simulink model "Copy_of_MPC_control"  (R2018a)
settings: Solver=FixedStepAuto  StartTime=0  StopTime=Tend  FixedStep=0.001  RelTol=5e-3
model workspace (MAT data in the model file):
  A_mu = 10
  B_reff = 8.386
  Cz = 7766.25
  DCT_Param : struct (value not decoded)
  D_reff = 0.25826
  Downshift_Speeds = [9.5625 12.9375 16.3125 19.6875 23.0625 26.4375 29.8125 33.1875 36.5625 39.9375 43.3125 46.6875 ... (28 elements, 4x7)]
  Pedal_Positions = [0.1 0.4 0.5 0.9]
  SUS : struct (value not decoded)
  Upshift_Speeds = [12.9375 16.3125 19.6875 33 26.4375 29.8125 33.1875 52.5 39.9375 43.3125 46.6875 77.25 ... (28 elements, 4x7)]
  VEH : struct (value not decoded)
  V_o = 16.7
  V_xlow = 1
  WH : struct (value not decoded)
  a = 1.4
  alpha_max = 1.5
  alpha_min = -1.5
  b = 1.8
  c_zo = 209651
  epsilon = 0.1
  h = 0.134
  path : struct (value not decoded)
  pio = 220000
  q_Fcx = 0
  q_Fz2 = 15.4
  q_Fzy = 0
  q_reo = 0.9974
  q_sx1 = -0.007764
  q_sx10 = 0.2824
  q_sx11 = 5.349
  q_sx12 = 0
  q_sx13 = 0
  q_sx14 = 0
  q_sx2 = 1.1915
  q_sx3 = 0.013948
  q_sx4 = 4.912
  q_sx5 = 1.02
  q_sx6 = 22.83
  q_sx7 = 0.7104
  q_sx8 = -0.023393
  q_sx9 = 0.6581
  q_sy1 = 0.00702
  q_sy2 = 0
  q_sy3 = 0.001515
  q_sy4 = 8.514e-05
  q_sy5 = 0
  q_sy6 = 0
  q_sy7 = 0.9008
  q_sy8 = -0.4089
  q_v1 = 0.0007742
  q_v2 = 0.04667
  r_Bx1 = 12.531
  r_Bx2 = 9.532
  r_Bx3 = 0
  r_By1 = 10.615
  r_By2 = 7.705
  r_By3 = 3.433e-06
  r_By4 = 0
  r_Cx1 = 1.019
  r_Cy1 = 1.0585
  r_Ex1 = -0.4487
  r_Ex2 = -0.4726
  r_Ey1 = 0.3132
  r_Ey2 = 7.63e-06
  r_Hx1 = 0.0002374
  r_Hy1 = 0.011646
  r_Hy2 = 7.63e-06
  r_Vy1 = 0.05654
  r_Vy2 = 7.63e-06
  r_Vy3 = 0
  r_Vy4 = 99.9
  r_Vy5 = 2
  r_Vy6 = 15.814
  r_o = 0.3135
  vehWidth = 2
  w = 1
symbols that are objects in the model workspace (value not decoded): VEH
undefined symbols (not defined in the file): C_Brake, C_Final, C_Front, C_Front_1, C_Front_2, C_Middle, C_out_Brake, C_out_Final, C_out_Front, C_out_Front_1, C_out_Front_2, C_out_Middle, Co, Cok_Brake, Cok_Final, Cok_Front_1, Cok_Front_2, Cok_Middle, Cso, D_out_Brake, D_out_Final, D_out_Front, D_out_Front_1, D_out_Front_2, D_out_Middle, Earlytochange, Earlytochange2, F, F_Brake, F_Final, F_Front, F_Front_1, F_Front_2, F_Middle, Fs, G_Brake, G_Final, G_Front_1, G_Front_2, G_Middle, G_sys_Brake, G_sys_Final, G_sys_Front, G_sys_Front_1, G_sys_Front_2, G_sys_Middle, Gd, Gd_Brake, Gd_Final, Gd_Front, Gd_Front_1, Gd_Front_2, Gd_Middle, Go, Gsd, Gso, H_Brake, H_Final, H_Front_1, H_Front_2 ... (+60)
libraries: simulink x10, sim3dlib x4, autolibutils x2, vehdynlibviscommon x2
(part 7 of 8)

== matlab function Copy_of_MPC_control/observer/simulator_1/VH2P/YV2P ==
  data: Velocity input; LastVelocity input; Yaw input; LastYaw input; Tsim input; LastTsim input; Lastpostion input; Position output
function Position  = YV2P(Velocity,LastVelocity, Yaw, LastYaw, Tsim, LastTsim, Lastpostion)
if Tsim >= 0.1
    Position = zeros(2,1);
    X0 = Lastpostion(1,:); Y0 = Lastpostion(2,:);
    Vx0 = [LastVelocity*cos(LastYaw); Velocity*cos(Yaw)];
    Vy0 = [LastVelocity*sin(LastYaw); Velocity*sin(Yaw)];
    Yaw_sim = [LastYaw; Yaw];
    T =[LastTsim; Tsim];
    [ X_tmp, Y_tmp] = YV2P( T, X0, Y0, Vx0, Vy0, Yaw_sim, zeros(2,1) );
    Position = [X_tmp(end,:); Y_tmp(end,:)];
else
    Position = [0; 0];
end
end

== matlab function Copy_of_MPC_control/observer/observer_2/gate ==
  data: select_overlap input; state output
function state = gate(select_overlap)
if select_overlap == 2
    state = 1;
else
    state = 0;
end
end

== matlab function Copy_of_MPC_control/observer/simulator_3/VH2P/YV2P ==
  data: Velocity input; LastVelocity input; Yaw input; LastYaw input; Tsim input; LastTsim input; Lastpostion input; Position output
function Position  = YV2P(Velocity,LastVelocity, Yaw, LastYaw, Tsim, LastTsim, Lastpostion)
if Tsim >= 0.1
    Position = zeros(2,1);
    X0 = Lastpostion(1,:); Y0 = Lastpostion(2,:);
    Vx0 = [LastVelocity*cos(LastYaw); Velocity*cos(Yaw)];
    Vy0 = [LastVelocity*sin(LastYaw); Velocity*sin(Yaw)];
    Yaw_sim = [LastYaw; Yaw];
    T =[LastTsim; Tsim];
    [ X_tmp, Y_tmp] = YV2P( T, X0, Y0, Vx0, Vy0, Yaw_sim, zeros(2,1) );
    Position = [X_tmp(end,:); Y_tmp(end,:)];
else
    Position = [0; 0];
end
end

== matlab function Copy_of_MPC_control/observer/simulator_2/Mpc_Simulator_Middle/MATLAB Function ==
  data: r output; JE input; phi input; Fxh input; Qc input; U output; M input; Np input; Heading_updated input; Velocity_updated input; Rs input; Tsim input; select_MPC input; U_delay input
function [r,U] = HQP(JE ,phi,Fxh ,Qc ,M ,Np,Heading_updated ,Velocity_updated ,Rs ,Tsim, select_MPC,U_delay)
u1_max =  5/3*pi; u1_min = -5/3*pi;
u2_max =  1; u2_min = -1;
du1_inc =  1*5/3*pi;du1_dec =  1*5/3*pi;
du2_inc =  1;du2_dec =  1;
U_max = []; U_min = [];
for i = 1:Np
    U_max = [U_max; [u1_max; u2_max]];
    U_min = [U_min; [-u1_min; -u2_min]];
end

dU_plus = []; dU_minus = [];
for i = 1:Np
    dU_plus = [dU_plus; [U_delay(1) + du1_inc; U_delay(2) + du2_inc]];
    dU_minus = [dU_minus; [-U_delay(1) + du1_dec; -U_delay(2) + du2_dec;]];
end
N = [U_max;
      U_min;
      dU_plus;
      dU_minus;          
     ];
if Tsim > 0 && select_MPC ~= 5
    for i = 1: Np
        Rs(2*i,:) = Heading_updated(i,:);
        Rs(2*i-1,:) = Velocity_updated(i,:);
    end
end
JF = -2*phi'*Qc*(Rs-Fxh);
[u,lambda]= HQP(JE,JF,M,N);
U = u(1:2);
r = Rs(1:2,:);
end

== matlab function Copy_of_MPC_control/YV_update/MATLAB Function2 ==
  data: XYplot_ref input; Velocity_updated output; XYplot_sim input; Velocity_sim input; Yaw_sim input; Ts input; Tsim input; Heading_updated output
function [Velocity_updated, Heading_updated] = VY_update(XYplot_ref, XYplot_sim, Velocity_sim, Yaw_sim, Ts, Tsim)
Np = 6;
Heading_updated = zeros(Np,1); Velocity_updated = zeros(Np,1);
coder.extrinsic('P2YV');
T = []; 
for j = 1:Np+1
    T = [T; Tsim+(j-1)*Ts];
end
X = [];
for i = 1:Np
    X = [X; XYplot_ref(2*i-1,:)];
end
Y = [];
for i = 1:Np
    Y = [Y; XYplot_ref(2*i,:)];
end

X = [XYplot_sim(1,:); X];
Y = [XYplot_sim(2,:); Y];   
Vx0 = Velocity_sim*cos(Yaw_sim);
Vy0 = Velocity_sim*sin(Yaw_sim);
Yaw0 = Yaw_sim;

[Velocity_updated, Heading_updated] = P2YV(0,0, T , X , Y , Vx0 , Vy0 , Yaw0, Np, 0, 0 );
end

== matlab function Copy_of_MPC_control/observer/simulator_2/VH2P/YV2P ==
  data: Velocity input; LastVelocity input; Yaw input; LastYaw input; Tsim input; LastTsim input; Lastpostion input; Position output
function Position  = YV2P(Velocity,LastVelocity, Yaw, LastYaw, Tsim, LastTsim, Lastpostion)
if Tsim >= 0.1
    Position = zeros(2,1);
    X0 = Lastpostion(1,:); Y0 = Lastpostion(2,:);
    Vx0 = [LastVelocity*cos(LastYaw); Velocity*cos(Yaw)];
    Vy0 = [LastVelocity*sin(LastYaw); Velocity*sin(Yaw)];
    Yaw_sim = [LastYaw; Yaw];
    T =[LastTsim; Tsim];
    [ X_tmp, Y_tmp] = YV2P( T, X0, Y0, Vx0, Vy0, Yaw_sim, zeros(2,1) );
    Position = [X_tmp(end,:); Y_tmp(end,:)];
else
    Position = [0; 0];
end
end

== matlab function Copy_of_MPC_control/observer/simulator_2/VH2P/gate ==
  data: select_overlap input; state output
function state = gate(select_overlap)
if select_overlap == 2
    state = 1;
else
    state = 0;
end
end

== matlab function Copy_of_MPC_control/Controllers/ECU/MATLAB Function ==
  data: input output; input input; output output
function [input,output] = debug(input)
if isnan(input) || isinf(input)
    output = 1;
    input = 0;
else
    output = 0;
    input = input;
end
end

== matlab function Copy_of_MPC_control/observer123/Final Observer2/Subsystem/Mpc_Simulator_Final/MATLAB Function ==
  data: Upd_flag input; Timetochange input; Ref output; JE input; U output; M input; Np input; phi input; Qc input; Fxh input; Yup input; Vup input; Rs input; Rs_V input; Tsim input; Upd_end input; u input
function [Ref,U] = HQP(Upd_flag, Timetochange,JE,M,Np,phi,Qc,Fxh,Yup,Vup,Rs,Rs_V,Tsim,Upd_end,u)

% if Tsim < 6.27 %(sec)
%     u1_max =  5/3*pi; u1_min = -5/3*pi;
%     u2_max =  0.3; u2_min = -1;
%     du1_inc =  1*5/3*pi; 
%     du1_dec =  1*5/3*pi; 
%     du2_inc =  0.03;
%     du2_dec =  0.03;
% else 
    u1_max =  5/3*pi; u1_min = -5/3*pi;
    u2_max =  1; u2_min = -1;
    du1_inc =  1*5/3*pi;
    du1_dec =  1*5/3*pi;
    du2_inc =  1;
    du2_dec =  1;
% end
% du1_max =  0.1*abs(Fxh(1,:)); 
% du2_max =  0.05*abs(Fxh(1,:)); 
% Y1_min = Rs(1,:) - 2;%V
% Y1_max = Rs(1,:) + 2;%V
% Y2_min = Rs(2,:) - 0.2;%Y
% Y2_max = Rs(2,:) + 0.2;%Y
% 
% Y1_min = -10;%V
% Y2_min = -100;%Y
% Y1_max = 50;%V
% Y2_max = 100;%Y

% Y_max = [];
% Y_min = [];
% for i = 1:Np
%     Y_max = [Y_max;[Y1_max;Y2_max]];
%     Y_min = [Y_min;[Y1_min;Y2_min]];
% end

U_max = []; U_min = [];
for i = 1:Np
    U_max = [U_max; [u1_max; u2_max]];
    U_min = [U_min; [-u1_min; -u2_min]];
end

dU_plus = []; dU_minus = [];
for i = 1:Np
    dU_plus = [dU_plus; [u(1) + du1_inc; u(2) + du2_inc]];
    dU_minus = [dU_minus; [-u(1) + du1_dec; -u(2) + du2_dec;]];
end
rr = [U_max;
      U_min;
      dU_plus;
      dU_minus;          
     ];
 
% rr_y = [Y_max - Fxh;
%        -Y_min + Fxh;
%        ];
N = [];
N = rr; 
% N = [rr;rr_y];


if Tsim > 0 && Tsim < Upd_end
    for i = 1: Np
        Rs(2*i,:) = Yup(i,:);
        Rs(2*i-1,:) = Vup(i,:);
    end
% elseif Tsim >= 65
%     for i = 1: Np
%         Rs(2*i,:) = Yup(i,:);
% %         Rs(2*i-1,:) = Vup(i,:);
%     end
end


JF = -2*phi'*Qc*(Rs-Fxh);
[uc,lambda]= HQP(JE,JF,M,N);
U = uc(1:2);
% if Tsim <= Timetochange
%     U(1,:) = 1e-9;
% end
Ref = Rs(1:2,:);
% lambda
end

== matlab function Copy_of_MPC_control/observer/simulator_2/YV_update_Np/MATLAB Function2 ==
  data: XYplot_ref input; Velocity_updated output; XYplot_sim input; Velocity_sim input; Yaw_sim input; Ts input; Tsim input; Heading_updated output
function [Velocity_updated, Heading_updated] = VY_update(XYplot_ref, XYplot_sim, Velocity_sim, Yaw_sim, Ts, Tsim)
Np = 6;
 disp(sprintf('Simulation time : %2.1f sec',Tsim)) 
 Heading_updated = zeros(Np,1); Velocity_updated = zeros(Np,1);
coder.extrinsic('P2YV');
T = []; 
for j = 1:Np+1
    T = [T; Tsim+(j-1)*Ts];
end
X = [];
for i = 1:Np
    X = [X; XYplot_ref(2*i-1,:)];
end
Y = [];
for i = 1:Np
    Y = [Y; XYplot_ref(2*i,:)];
end

X = [XYplot_sim(1,:); X];
Y = [XYplot_sim(2,:); Y];   
Vx0 = Velocity_sim*cos(Yaw_sim);
Vy0 = Velocity_sim*sin(Yaw_sim);
Yaw0 = Yaw_sim;

[Velocity_updated, Heading_updated] = P2YV(0,0, T , X , Y , Vx0 , Vy0 , Yaw0, Np, 0, 0 );
end

== matlab function Copy_of_MPC_control/observer/simulator_2/gate ==
  data: select_overlap input; state output
function state = gate(select_overlap)
if select_overlap == 2
    state = 1;
else
    state = 0;
end
end

== stateflow chart Copy_of_MPC_control/all_system/Controllers1/Transmission Controller/TCM/TCM Shift Controller ==
  settings: sampleTime=0.01
  state GearState [parallel]
    settings: executionOrder=1
    state Neutral
      en:
      GearState = 0;
    state G1
      en:
      GearState = 1;
    state G2
      en:
      GearState = 2;
      du:
      [SpdThr] = calc(2,pedal,speed);
    state G3
      en:
      GearState = 3;
      du:
      [SpdThr] = calc(3,pedal,speed);
    state G8
      en:
      GearState = 8;
    state G7
      en:
      GearState = 7;
    state G6
      en:
      GearState = 6;
    state G5
      en:GearState=5;
      du:[SpdThr]=calc(5,pedal,speed);
    state G4
      en:
      GearState = 4;
      du:
      [SpdThr] = calc(4,pedal,speed);
    (default) -> G1
    Neutral -> G1 : [~Neutral]
    G1 -> G2 [order 1] : Up
    G2 -> G3 [order 1] : Up
    G1 -> Neutral [order 2] : [Neutral]
    G2 -> G1 [order 2] : Down
    G3 -> G2 [order 2] : Down
    G3 -> G4 [order 1] : Up
    G4 -> G3 [order 2] : Down
    G7 -> G8 [order 1] : Up
    G5 -> G6 [order 1] : Up
    G6 -> G7 [order 1] : Up
    G4 -> G5 [order 1] : Up
    G5 -> G4 [order 2] : Down
    G6 -> G5 [order 2] : Down
    G7 -> G6 [order 2] : Down
    G8 -> G7 : Down
  state SelectionState [parallel]
    du:[up_th]=calc_up(GearState,pedal);
    du:[down_th]=calc_down(GearState,pedal);
    settings: executionOrder=2
    state SteadyState
      en:
      clutchControl = 0;
    state preDownShifting
    state preUpShifting
    state UpShifting
      en:
      GearState = GearState + 0.5;
    state DownShifting
      en:
      GearState = GearState - 0.5;
    (default) -> SteadyState
    SteadyState -> (junction 62) [order 1] : [speed < down_th && ...
        | GearState >1]
    SteadyState -> (junction 128) [order 2] : [speed > up_th &&...
        | GearState <= 5 && ...
        | floor(GearState) == GearState]
    (junction 62) -> preDownShifting
    (junction 128) -> preUpShifting
    (junction 168) -> SteadyState
    (junction 23) -> SteadyState
    (junction 161) -> SteadyState
    preDownShifting -> (junction 168) [order 2] : [speed >= down_th]
    preUpShifting -> (junction 161) [order 2] : [speed <= up_th]
    preUpShifting -> UpShifting [order 1] : after(0.5,sec)
        | [speed>up_th]
    preDownShifting -> DownShifting [order 1] : after(0.5, sec)
        | [speed < down_th - 2]
    DownShifting -> (junction 23) : {GearState.Down;}
    UpShifting -> (junction 23) : {GearState.Up;}
  state up_th = calc_up(gear,pedal) [function]
  state down_th = calc_down(gear,pedal) [function]
  state SpdThr = calc(gear,pedal,speed) [function]
  data: gear function_input; pedal function_input; up_th function_output; gear function_input; pedal function_input; down_th function_output; gear function_input; pedal function_input; SpdThr function_output; speed function_input; GearState output int8; speed input; pedal input; clutchControl local double; SpdThr local double; Neutral input; up_th local double; down_th local double
  events: Up local EITHER_EDGE_EVENT; Down local EITHER_EDGE_EVENT

== matlab function Copy_of_MPC_control/all_system/Dataselect1/Dataselect ==
  data: timing input; select output; Statechange input; Statechange2 input
function select = Dataselect(timing,Statechange,Statechange2)    
    if timing < Statechange
        select = 1;
    elseif timing < Statechange2
        select = 2;
    else 
        select = 3;
    end
end

== matlab function Copy_of_MPC_control/all_system/Final Observer2/Subsystem/Mpc_Simulator_Final/MATLAB Function ==
  data: Upd_flag input; Timetochange input; Ref output; JE input; U output; M input; Np input; phi input; Qc input; Fxh input; Yup input; Vup input; Rs input; Rs_V input; Tsim input; Upd_end input; u input
function [Ref,U] = HQP(Upd_flag, Timetochange,JE,M,Np,phi,Qc,Fxh,Yup,Vup,Rs,Rs_V,Tsim,Upd_end,u)

% if Tsim < 6.27 %(sec)
%     u1_max =  5/3*pi; u1_min = -5/3*pi;
%     u2_max =  0.3; u2_min = -1;
%     du1_inc =  1*5/3*pi; 
%     du1_dec =  1*5/3*pi; 
%     du2_inc =  0.03;
%     du2_dec =  0.03;
% else 
    u1_max =  5/3*pi; u1_min = -5/3*pi;
    u2_max =  1; u2_min = -1;
    du1_inc =  1*5/3*pi;
    du1_dec =  1*5/3*pi;
    du2_inc =  1;
    du2_dec =  1;
% end
% du1_max =  0.1*abs(Fxh(1,:)); 
% du2_max =  0.05*abs(Fxh(1,:)); 
% Y1_min = Rs(1,:) - 2;%V
% Y1_max = Rs(1,:) + 2;%V
% Y2_min = Rs(2,:) - 0.2;%Y
% Y2_max = Rs(2,:) + 0.2;%Y
% 
% Y1_min = -10;%V
% Y2_min = -100;%Y
% Y1_max = 50;%V
% Y2_max = 100;%Y

% Y_max = [];
% Y_min = [];
% for i = 1:Np
%     Y_max = [Y_max;[Y1_max;Y2_max]];
%     Y_min = [Y_min;[Y1_min;Y2_min]];
% end

U_max = []; U_min = [];
for i = 1:Np
    U_max = [U_max; [u1_max; u2_max]];
    U_min = [U_min; [-u1_min; -u2_min]];
end

dU_plus = []; dU_minus = [];
for i = 1:Np
    dU_plus = [dU_plus; [u(1) + du1_inc; u(2) + du2_inc]];
    dU_minus = [dU_minus; [-u(1) + du1_dec; -u(2) + du2_dec;]];
end
rr = [U_max;
      U_min;
      dU_plus;
      dU_minus;          
     ];
 
% rr_y = [Y_max - Fxh;
%        -Y_min + Fxh;
%        ];
N = [];
N = rr; 
% N = [rr;rr_y];


if Tsim > 0 && Tsim < Upd_end
    for i = 1: Np
        Rs(2*i,:) = Yup(i,:);
        Rs(2*i-1,:) = Vup(i,:);
    end
% elseif Tsim >= 65
%     for i = 1: Np
%         Rs(2*i,:) = Yup(i,:);
% %         Rs(2*i-1,:) = Vup(i,:);
%     end
end


JF = -2*phi'*Qc*(Rs-Fxh);
[uc,lambda]= HQP(JE,JF,M,N);
U = uc(1:2);
% if Tsim <= Timetochange
%     U(1,:) = 1e-9;
% end
Ref = Rs(1:2,:);
% lambda
end

== matlab function Copy_of_MPC_control/all_system/Final Observer2/Subsystem/Pose updete k/Update ==
  settings: updateMethod=DISCRETE  sampleTime=Ts
  data: Rs_V_now input; Rs_Y_now input; XYline input; XYplot input; XYplot_sim input; Last_XYplot_sim input; Velocity_sim input; Last_Velocity_sim input; Heading_sim input; Last_Heading_sim input; Tsim input; Last_Heading_end input; Velocity_updated output; Heading_updated output [1..5]; Heading_end output
function [Velocity_updated, Heading_updated, Heading_end] = Y_update(Rs_V_now, Rs_Y_now, ...
        XYline, XYplot, XYplot_sim, Last_XYplot_sim, Velocity_sim, Last_Velocity_sim, Heading_sim, Last_Heading_sim, ... 
    Tsim, Last_Heading_end)
    disp(sprintf('Simulation time : %2.1f sec',Tsim)) 
    Np = 5; Ts = 0.1;
    Heading_updated = zeros(Np,1); Velocity_updated = zeros(Np,1);Heading_end = 0;
    coder.extrinsic('intersections');
    coder.extrinsic('P2YV');
%     coder.varsize('Velocity_updated_tmp',[5 1]);
%     coder.varsize('Heading_updated_tmp',[5 1]);
     if Tsim == 0 
        plot(XYline(:,2),XYline(:,1),'black');
    end
   

%%Create half-circle    

    N = 30;
    theta = zeros(Np-1,N+1); Veh_circle = zeros(N+1,(Np-1)*2); 
    xp = zeros(1,N+1); yp = zeros(1,N+1); X = [];  Y = []; X_tmp = 0; Y_tmp = 0;
    lookahead = zeros(Np-1,1);
    
    XYplot_sim_tmp = XYplot_sim;    

%     if Velocity_sim > 0.5
        Velocity_ahead = [Velocity_sim; Rs_V_now(2:Np-1,:)];
%     else
%         Velocity_ahead = Rs_V_now;
%     end

    lookahead = Velocity_ahead*Ts;
    Headngahead = [Heading_sim; Rs_Y_now(2:Np-1,:)];
%     lookahead = [1; 1.5; 2; 2.5; 3];
        
    for j = 1:Np-1        
        theta = Headngahead(j,:)-pi/4 : pi/2/N : Headngahead(j,:)+pi/4;
        xp = lookahead(j,:)*cos(theta) + XYplot_sim_tmp(1,:)*ones(1,length(theta));
        yp = lookahead(j,:)*sin(theta) + XYplot_sim_tmp(2,:)*ones(1,length(theta));
        Veh_circle(:,2*j-1:2*j) = [xp' yp'];
       
    %Find the intersection    
         
        [X_tmp, Y_tmp] = intersections(XYplot(:,1), XYplot(:,2), Veh_circle(:,2*j-1), Veh_circle(:,2*j),0); 
        
        if X_tmp == 0 && Y_tmp == 0
%             X = X_tmp(1:j-1,:);
%             Y = Y_tmp(1:j-1,:);
            break;
        end

        X = [X; X_tmp];
        Y = [Y; Y_tmp];   
        XYplot_sim_tmp = [X_tmp; Y_tmp];
        
    end 
    
%%Obtain predict Velocity and Heading angle
   
  
    
    X = [Last_XYplot_sim(1,:); XYplot_sim(1,:); X];
    Y = [Last_XYplot_sim(2,:); XYplot_sim(2,:); Y];
    Vx0 = Last_Velocity_sim*cos(Last_Heading_sim);
    Vy0 = Last_Velocity_sim*sin(Last_Heading_sim);
    Yaw0 = Last_Heading_sim;
     
    T_sample = []; 
    for j = 1:length(X)
        T_sample = [T_sample; Tsim+(j-1)*Ts];
    end
    
   [Velocity_updated, Heading_updated] = P2YV(0, T_sample , X , Y , Vx0 , Vy0 , Yaw0, Np, Last_Heading_end );
   Heading_end = Heading_updated(end,:);

%     Heading_tmp_end = atan2(XYplot(end,2)-XYplot_sim(2,:), XYplot(end,1)-XYplot_sim(1,:));
% 
%     if  ((Heading_tmp_end - Heading_tmp_end_delay) < -5/3*pi) % Angle compensation
%         Heading_flag_end = Heading_flag_end + 1;
%     elseif ((Heading_tmp_end - Heading_tmp_end_delay) > 5/3*pi)
%         Heading_flag_end = Heading_flag_end - 1;
%     end
%     
%     if flag == 1
%         Heading_updated(1:end) = Heading_tmp_end + Heading_flag_end*2*pi;
%     end
%     if Tsim == 1.5
%         figure();
%         plot(XYplot(:,2),XYplot(:,1),'black-');
%         hold on;
%         plot(XYplot_sim(2,:),XYplot_sim(1,:),'b o');
%         plot(Veh_circle(:,2), Veh_circle(:,1),'b-');
%         plot(Veh_circle(:,4), Veh_circle(:,3),'b-');
%         plot(Veh_circle(:,6), Veh_circle(:,5),'b-');
%         plot(Veh_circle(:,8), Veh_circle(:,7),'b-');
%         plot(Veh_circle(:,10), Veh_circle(:,9),'b-');
%         plot(Y, X,'r x');
%     end

end

== matlab function Copy_of_MPC_control/all_system/Final Observer2/Subsystem/VH2P/YV2P ==
  data: Velocity input; Yaw input; LastVelocity input; LastYaw input; Tsim input; LastTsim input; Lastpostion input; Position output
function Position  = YV2P(Velocity, Yaw,  LastVelocity, LastYaw, Tsim, LastTsim, Lastpostion)
if Tsim >= 0.1
    Position = zeros(2,1);
    X0 = Lastpostion(1,:); Y0 = Lastpostion(2,:);
    Vx = [LastVelocity*cos(LastYaw); Velocity*cos(Yaw)];
    Vy = [LastVelocity*sin(LastYaw); Velocity*sin(Yaw)];
    Yaw_sim = [LastYaw; Yaw];
    T_sample =[LastTsim; Tsim];
    [ X_tmp, Y_tmp] = YV2P( T_sample, X0, Y0, Vx, Vy, Yaw_sim, zeros(2,1) );
    Position = [X_tmp(end,:); Y_tmp(end,:)];
else
    Position = [0; 0];
end

end

== matlab function Copy_of_MPC_control/all_system/Final Observer2/Subsystem/YV_update_Np/MATLAB Function2 ==
  data: XY_ref input; Velocity_updated output; XY_sim input; LastXY_sim input; Velocity_sim input; LastVelocity_sim input; Yaw_sim input; LastYaw_sim input; Tsim input; Heading_updated output
function [Velocity_updated, Heading_updated] = VY_update(XY_ref, XY_sim, LastXY_sim, Velocity_sim, LastVelocity_sim, Yaw_sim, LastYaw_sim, Tsim)
    disp(sprintf('Simulation time : %2.1f sec',Tsim)) 
 Ts = 0.1;
% Np = 6;
 Np = 6;

 Heading_updated = zeros(Np,1); Velocity_updated = zeros(Np,1);
coder.extrinsic('P2YV');
% T_sample = [Tsim-0.01; Tsim; Tsim+0.01];
% X = [LastXY_sim(1); XY_sim(1); XY_ref(1,:)];
% Y = [LastXY_sim(2); XY_sim(2); XY_ref(2,:)];

% T_sample = [Tsim-0.01; Tsim; Tsim+0.01; Tsim+0.02];
% X = [LastXY_sim(1); XY_sim(1); XY_ref(1,:); XY_ref(3,:)];
% Y = [LastXY_sim(2); XY_sim(2); XY_ref(2,:); XY_ref(4,:)];

T_sample = []; 
for j = 1:Np+1
    T_sample = [T_sample; Tsim+(j-1)*Ts];
end
X = [];
for i = 1:Np
    X = [X; XY_ref(2*i-1,:)];
end
Y = [];
for i = 1:Np
    Y = [Y; XY_ref(2*i,:)];
end

X = [XY_sim(1,:); X];
Y = [XY_sim(2,:); Y];   
Vx0 = Velocity_sim*cos(Yaw_sim);
Vy0 = Velocity_sim*sin(Yaw_sim);
Yaw0 = Yaw_sim;

[Velocity_updated, Heading_updated] = P2YV(0,0, T_sample , X , Y , Vx0 , Vy0 , Yaw0, Np, 0, 0 );

end

== matlab function Copy_of_MPC_control/all_system/Final_simulator1/Mpc_Simulator_Final/MATLAB Function ==
  data: Ref output; JE input; U output; M input; Np input; phi input; Qc input; Fxh input; Yup input; Vup input; Rs input; Rs_V input; Tsim input; Upd_end input; u input; lambda output
function [Ref,U,lambda] = HQP(JE,M,Np,phi,Qc,Fxh,Yup,Vup,Rs,Rs_V,Tsim,Upd_end,u)

% if Tsim < 6.27 %(sec)
%     u1_max =  5/3*pi; u1_min = -5/3*pi;
%     u2_max =  0.3; u2_min = -1;
%     du1_inc =  1*5/3*pi; 
%     du1_dec =  1*5/3*pi; 
%     du2_inc =  0.03;
%     du2_dec =  0.03;
% else 
    u1_max =  5/3*pi; u1_min = -5/3*pi;
    u2_max =  1; u2_min = -1;
    du1_inc =  1*5/3*pi;
    du1_dec =  1*5/3*pi;
    du2_inc =  1;
    du2_dec =  1;
% end
% du1_max =  0.1*abs(Fxh(1,:)); 
% du2_max =  0.05*abs(Fxh(1,:)); 
% Y1_min = Rs(1,:) - 2;%V
% Y1_max = Rs(1,:) + 2;%V
% Y2_min = Rs(2,:) - 0.2;%Y
% Y2_max = Rs(2,:) + 0.2;%Y
% 
% Y1_min = -10;%V
% Y2_min = -100;%Y
% Y1_max = 50;%V
% Y2_max = 100;%Y

% Y_max = [];
% Y_min = [];
% for i = 1:Np
%     Y_max = [Y_max;[Y1_max;Y2_max]];
%     Y_min = [Y_min;[Y1_min;Y2_min]];
% end

U_max = []; U_min = [];
for i = 1:Np
    U_max = [U_max; [u1_max; u2_max]];
    U_min = [U_min; [-u1_min; -u2_min]];
end

dU_plus = []; dU_minus = [];
for i = 1:Np
    dU_plus = [dU_plus; [u(1) + du1_inc; u(2) + du2_inc]];
    dU_minus = [dU_minus; [-u(1) + du1_dec; -u(2) + du2_dec;]];
end
rr = [U_max;
      U_min;
      dU_plus;
      dU_minus;          
     ];
 
% rr_y = [Y_max - Fxh;
%        -Y_min + Fxh;
%        ];
N = [];
N = rr; 
% N = [rr;rr_y];

if Tsim > 0 && Tsim < Upd_end
% if Tsim > 0.2
    for i = 1: Np
        Rs(2*i,:) = Yup(i,:);
        Rs(2*i-1,:) = Vup(i,:);
    end
end

JF = -2*phi'*Qc*(Rs-Fxh);
[uc,lambda]= HQP(JE,JF,M,N);
U = uc(1:2);
Ref = Rs(1:2,:);
% lambda
end

== matlab function Copy_of_MPC_control/all_system/Final_simulator1/VH2P/Trigger/Trigger ==
  data: timing input; Trigger output; Earlytochange2 input
function Trigger = initial_position_trigger(timing,Earlytochange2)
Trigger = 0;    
    if timing == Earlytochange2
        Trigger = 1;
    end
end

== matlab function Copy_of_MPC_control/all_system/Final_simulator1/VH2P/YV2P ==
  data: Velocity input; Yaw input; LastVelocity input; LastYaw input; Tsim input; LastTsim input; Lastpostion input; Position output
function Position  = YV2P(Velocity, Yaw,  LastVelocity, LastYaw, Tsim, LastTsim, Lastpostion)
if Tsim >= 0.1
    Position = zeros(2,1);
    X0 = Lastpostion(1,:); Y0 = Lastpostion(2,:);
    Vx = [LastVelocity*cos(LastYaw); Velocity*cos(Yaw)];
    Vy = [LastVelocity*sin(LastYaw); Velocity*sin(Yaw)];
    Yaw_sim = [LastYaw; Yaw];
    T_sample =[LastTsim; Tsim];
    [ X_tmp, Y_tmp] = YV2P( T_sample, X0, Y0, Vx, Vy, Yaw_sim, zeros(2,1) );
    Position = [X_tmp(end,:); Y_tmp(end,:)];
else
    Position = [0; 0];
end

end

== matlab function Copy_of_MPC_control/all_system/Final_simulator1/YV_update_Np/MATLAB Function2 ==
  data: XY_ref input; Velocity_updated output; XY_sim input; LastXY_sim input; Velocity_sim input; LastVelocity_sim input; Yaw_sim input; LastYaw_sim input; Tsim input; Heading_updated output
function [Velocity_updated, Heading_updated] = VY_update(XY_ref, XY_sim, LastXY_sim, Velocity_sim, LastVelocity_sim, Yaw_sim, LastYaw_sim, Tsim)
    disp(sprintf('Simulation time : %2.1f sec',Tsim)) 
 Ts = 0.1;
%  Np = 6;
 Np = 6;

 Heading_updated = zeros(Np,1); Velocity_updated = zeros(Np,1);
coder.extrinsic('P2YV_Simulator');
% T_sample = [Tsim-0.01; Tsim; Tsim+0.01];
% X = [LastXY_sim(1); XY_sim(1); XY_ref(1,:)];
% Y = [LastXY_sim(2); XY_sim(2); XY_ref(2,:)];

% T_sample = [Tsim-0.01; Tsim; Tsim+0.01; Tsim+0.02];
% X = [LastXY_sim(1); XY_sim(1); XY_ref(1,:); XY_ref(3,:)];
% Y = [LastXY_sim(2); XY_sim(2); XY_ref(2,:); XY_ref(4,:)];

T_sample = []; 
for j = 1:Np+1
    T_sample = [T_sample; Tsim+(j-1)*Ts];
end
X = [];
for i = 1:Np
    X = [X; XY_ref(2*i-1,:)];
end
Y = [];
for i = 1:Np
    Y = [Y; XY_ref(2*i,:)];
end

X = [XY_sim(1,:); X];
Y = [XY_sim(2,:); Y];   
Vx0 = Velocity_sim*cos(Yaw_sim);
Vy0 = Velocity_sim*sin(Yaw_sim);
Yaw0 = Yaw_sim;

[Velocity_updated, Heading_updated] = P2YV_Simulator(0,0, T_sample , X , Y , Vx0 , Vy0 , Yaw0, Np, 0, 0 );

end

== matlab function Copy_of_MPC_control/all_system/Final_simulator_ operating_time1/MATLAB Function2 ==
  data: timing input; state output; Earlytochange2 input
function state = OperatingtimeFinal(timing,Earlytochange2)
    if timing >= Earlytochange2
        state = 1;
    else
        state = 0;
    end
end

== matlab function Copy_of_MPC_control/all_system/Front_simulator1/Mpc_Simulator_Front/MATLAB Function ==
  data: Ref output; JE input; U output; M input; Np input; phi input; Qc input; Fxh input; Yup input; Vup input; Rs input; Rs_V input; Tsim input; u input; lambda output
function [Ref,U,lambda] = HQP(JE,M,Np,phi,Qc,Fxh,Yup,Vup,Rs,Rs_V,Tsim,u)

% if Tsim < 6.27 %(sec)
%     u1_max =  5/3*pi; u1_min = -5/3*pi;
%     u2_max =  0.3; u2_min = -1;
%     du1_inc =  1*5/3*pi; 
%     du1_dec =  1*5/3*pi; 
%     du2_inc =  0.03;
%     du2_dec =  0.03;
% else 
    u1_max =  5/3*pi; u1_min = -5/3*pi;
    u2_max =  1; u2_min = -1;
    du1_inc =  1*5/3*pi;
    du1_dec =  1*5/3*pi;
    du2_inc =  1;
    du2_dec =  1;
% end
% du1_max =  0.1*abs(Fxh(1,:)); 
% du2_max =  0.05*abs(Fxh(1,:)); 
% Y1_min = Rs(1,:) - 2;%V
% Y1_max = Rs(1,:) + 2;%V
% Y2_min = Rs(2,:) - 0.2;%Y
% Y2_max = Rs(2,:) + 0.2;%Y
% 
% Y1_min = -10;%V
% Y2_min = -100;%Y
% Y1_max = 50;%V
% Y2_max = 100;%Y

% Y_max = [];
% Y_min = [];
% for i = 1:Np
%     Y_max = [Y_max;[Y1_max;Y2_max]];
%     Y_min = [Y_min;[Y1_min;Y2_min]];
% end

U_max = []; U_min = [];
for i = 1:Np
    U_max = [U_max; [u1_max; u2_max]];
    U_min = [U_min; [-u1_min; -u2_min]];
end

dU_plus = []; dU_minus = [];
for i = 1:Np
    dU_plus = [dU_plus; [u(1) + du1_inc; u(2) + du2_inc]];
    dU_minus = [dU_minus; [-u(1) + du1_dec; -u(2) + du2_dec;]];
end
rr = [U_max;
      U_min;
      dU_plus;
      dU_minus;          
     ];
 
% rr_y = [Y_max - Fxh;
%        -Y_min + Fxh;
%        ];
N = [];
N = rr; 
% N = [rr;rr_y];

% if Tsim > 0.2
    for i = 1: Np
        Rs(2*i,:) = Yup(i,:);
        Rs(2*i-1,:) = Vup(i,:);
    end
% end

JF = -2*phi'*Qc*(Rs-Fxh);
[uc,lambda]= HQP(JE,JF,M,N);
U = uc(1:2);
Ref = Rs(1:2,:);
% lambda
end

== matlab function Copy_of_MPC_control/all_system/Front_simulator1/VH2P/YV2P ==
  data: Velocity input; Yaw input; LastVelocity input; LastYaw input; Tsim input; LastTsim input; Lastpostion input; Position output
function Position  = YV2P(Velocity, Yaw,  LastVelocity, LastYaw, Tsim, LastTsim, Lastpostion)
if Tsim >= 0.1
    Position = zeros(2,1);
    X0 = Lastpostion(1,:); Y0 = Lastpostion(2,:);
    Vx = [LastVelocity*cos(LastYaw); Velocity*cos(Yaw)];
    Vy = [LastVelocity*sin(LastYaw); Velocity*sin(Yaw)];
    Yaw_sim = [LastYaw; Yaw];
    T_sample =[LastTsim; Tsim];
    [ X_tmp, Y_tmp] = YV2P( T_sample, X0, Y0, Vx, Vy, Yaw_sim, zeros(2,1) );
    Position = [X_tmp(end,:); Y_tmp(end,:)];
else
    Position = [0; 0];
end

end

== matlab function Copy_of_MPC_control/all_system/Front_simulator1/YV_update_Np/MATLAB Function2 ==
  data: XY_ref input; Velocity_updated output; XY_sim input; LastXY_sim input; Velocity_sim input; LastVelocity_sim input; Yaw_sim input; LastYaw_sim input; Tsim input; Heading_updated output
function [Velocity_updated, Heading_updated] = VY_update(XY_ref, XY_sim, LastXY_sim, Velocity_sim, LastVelocity_sim, Yaw_sim, LastYaw_sim, Tsim)
    disp(sprintf('Simulation time : %2.1f sec',Tsim)) 
 Ts = 0.1;
%  Np = 6;
 Np = 6;

 Heading_updated = zeros(Np,1); Velocity_updated = zeros(Np,1);
coder.extrinsic('P2YV_Simulator');
% T_sample = [Tsim-0.01; Tsim; Tsim+0.01];
% X = [LastXY_sim(1); XY_sim(1); XY_ref(1,:)];
% Y = [LastXY_sim(2); XY_sim(2); XY_ref(2,:)];

% T_sample = [Tsim-0.01; Tsim; Tsim+0.01; Tsim+0.02];
% X = [LastXY_sim(1); XY_sim(1); XY_ref(1,:); XY_ref(3,:)];
% Y = [LastXY_sim(2); XY_sim(2); XY_ref(2,:); XY_ref(4,:)];

T_sample = []; 
for j = 1:Np+1
    T_sample = [T_sample; Tsim+(j-1)*Ts];
end
X = [];
for i = 1:Np
    X = [X; XY_ref(2*i-1,:)];
end
Y = [];
for i = 1:Np
    Y = [Y; XY_ref(2*i,:)];
end

X = [XY_sim(1,:); X];
Y = [XY_sim(2,:); Y];   
Vx0 = Velocity_sim*cos(Yaw_sim);
Vy0 = Velocity_sim*sin(Yaw_sim);
Yaw0 = Yaw_sim;

[Velocity_updated, Heading_updated] = P2YV_Simulator(0,0, T_sample , X , Y , Vx0 , Vy0 , Yaw0, Np, 0, 0 );

end

== matlab function Copy_of_MPC_control/all_system/Front_simulator_ operating_time1/MATLAB Function1 ==
  data: timing input; state output; Statechange input
function state = OperatingtimeFront(timing,Statechange)
    if timing > Statechange
        state = 0;
    else
        state = 1;
    end
end

== matlab function Copy_of_MPC_control/all_system/MATLAB Function1 ==
  data: u input; Ac output; Br output
function [Ac, Br] = choose(u)
Ac = 0; Br = 0;
if u > 0 || u == 0
    Ac = u;
else
    Br = abs(u);
end
end

== matlab function Copy_of_MPC_control/all_system/Middle Observer2/Observer_state2/Observer_state2 ==
  data: timing input; state output; Timetochange input; Earlytochange input
function state = Observer_state2(timing,Timetochange,Earlytochange)
    if (timing <= Timetochange)
        state = 1;
    else
        state = 0;
    end
end

== matlab function Copy_of_MPC_control/all_system/Middle Observer2/Subsystem/Mpc_Simulator_Middle/MATLAB Function ==
  data: Upd_flag input; Timetochange input; Ref output; JE input; U output; M input; Np input; phi input; Qc input; Fxh input; Yup input; Vup input; Rs input; Rs_V input; Tsim input; Upd_end input; u input
function [Ref,U] = HQP(Upd_flag, Timetochange, JE,M,Np,phi,Qc,Fxh,Yup,Vup,Rs,Rs_V,Tsim,Upd_end,u)

% if Tsim < 6.27 %(sec)
%     u1_max =  5/3*pi; u1_min = -5/3*pi;
%     u2_max =  0.3; u2_min = -1;
%     du1_inc =  1*5/3*pi; 
%     du1_dec =  1*5/3*pi; 
%     du2_inc =  0.03;
%     du2_dec =  0.03;
% else 
    u1_max =  5/3*pi; u1_min = -5/3*pi;
    u2_max =  1; u2_min = -1;
    du1_inc =  1*5/3*pi;
    du1_dec =  1*5/3*pi;
    du2_inc =  1;
    du2_dec =  1;
% end
% du1_max =  0.1*abs(Fxh(1,:)); 
% du2_max =  0.05*abs(Fxh(1,:)); 
% Y1_min = Rs(1,:) - 2;%V
% Y1_max = Rs(1,:) + 2;%V
% Y2_min = Rs(2,:) - 0.2;%Y
% Y2_max = Rs(2,:) + 0.2;%Y
% 
% Y1_min = -10;%V
% Y2_min = -100;%Y
% Y1_max = 50;%V
% Y2_max = 100;%Y

% Y_max = [];
% Y_min = [];
% for i = 1:Np
%     Y_max = [Y_max;[Y1_max;Y2_max]];
%     Y_min = [Y_min;[Y1_min;Y2_min]];
% end

U_max = []; U_min = [];
for i = 1:Np
    U_max = [U_max; [u1_max; u2_max]];
    U_min = [U_min; [-u1_min; -u2_min]];
end

dU_plus = []; dU_minus = [];
for i = 1:Np
    dU_plus = [dU_plus; [u(1) + du1_inc; u(2) + du2_inc]];
    dU_minus = [dU_minus; [-u(1) + du1_dec; -u(2) + du2_dec;]];
end
rr = [U_max;
      U_min;
      dU_plus;
      dU_minus;          
     ];
 
% rr_y = [Y_max - Fxh;
%        -Y_min + Fxh;
%        ];
N = [];
N = rr; 
% N = [rr;rr_y];

if Tsim > 0 && Tsim < Upd_end
    for i = 1: Np
        Rs(2*i,:) = Yup(i,:);
        Rs(2*i-1,:) = Vup(i,:);
    end
% elseif Tsim >= 65
%     for i = 1: Np
%         Rs(2*i,:) = Yup(i,:);
% %         Rs(2*i-1,:) = Vup(i,:);
%     end
end


JF = -2*phi'*Qc*(Rs-Fxh);
[uc,lambda]= HQP(JE,JF,M,N);
U = uc(1:2);
% if Tsim <= Timetochange
%     U(1,:) = 1e-9;
% end
Ref = Rs(1:2,:);
% lambda
end

== matlab function Copy_of_MPC_control/all_system/Middle Observer2/Subsystem/Pose updete k/Update ==
  settings: updateMethod=DISCRETE  sampleTime=Ts
  data: Rs_V_now input; Rs_Y_now input; XYline input; XYplot input; XYplot_sim input; Last_XYplot_sim input; Velocity_sim input; Last_Velocity_sim input; Heading_sim input; Last_Heading_sim input; Tsim input; Last_Heading_end input; Velocity_updated output; Heading_updated output [1..5]; Heading_end output
function [Velocity_updated, Heading_updated, Heading_end] = Y_update(Rs_V_now, Rs_Y_now, ...
        XYline, XYplot, XYplot_sim, Last_XYplot_sim, Velocity_sim, Last_Velocity_sim, Heading_sim, Last_Heading_sim, ... 
    Tsim, Last_Heading_end)
    disp(sprintf('Simulation time : %2.1f sec',Tsim)) 
    Np = 5; Ts = 0.1;
    Heading_updated = zeros(Np,1); Velocity_updated = zeros(Np,1);Heading_end = 0;
    coder.extrinsic('intersections');
    coder.extrinsic('P2YV');
%     coder.varsize('Velocity_updated_tmp',[5 1]);
%     coder.varsize('Heading_updated_tmp',[5 1]);
     if Tsim == 0 
        plot(XYline(:,2),XYline(:,1),'black');
    end
   

%%Create half-circle    

    N = 30;
    theta = zeros(Np-1,N+1); Veh_circle = zeros(N+1,(Np-1)*2); 
    xp = zeros(1,N+1); yp = zeros(1,N+1); X = [];  Y = []; X_tmp = 0; Y_tmp = 0;
    lookahead = zeros(Np-1,1);
    
    XYplot_sim_tmp = XYplot_sim;    

%     if Velocity_sim > 0.5
        Velocity_ahead = [Velocity_sim; Rs_V_now(2:Np-1,:)];
%     else
%         Velocity_ahead = Rs_V_now;
%     end

    lookahead = Velocity_ahead*Ts;
    Headngahead = [Heading_sim; Rs_Y_now(2:Np-1,:)];
%     lookahead = [1; 1.5; 2; 2.5; 3];
        
    for j = 1:Np-1        
        theta = Headngahead(j,:)-pi/4 : pi/2/N : Headngahead(j,:)+pi/4;
        xp = lookahead(j,:)*cos(theta) + XYplot_sim_tmp(1,:)*ones(1,length(theta));
        yp = lookahead(j,:)*sin(theta) + XYplot_sim_tmp(2,:)*ones(1,length(theta));
        Veh_circle(:,2*j-1:2*j) = [xp' yp'];
       
    %Find the intersection    
         
        [X_tmp, Y_tmp] = intersections(XYplot(:,1), XYplot(:,2), Veh_circle(:,2*j-1), Veh_circle(:,2*j),0); 
        
        if X_tmp == 0 && Y_tmp == 0
%             X = X_tmp(1:j-1,:);
%             Y = Y_tmp(1:j-1,:);
            break;
        end

        X = [X; X_tmp];
        Y = [Y; Y_tmp];   
        XYplot_sim_tmp = [X_tmp; Y_tmp];
        
    end 
    
%%Obtain predict Velocity and Heading angle
   
  
    
    X = [Last_XYplot_sim(1,:); XYplot_sim(1,:); X];
    Y = [Last_XYplot_sim(2,:); XYplot_sim(2,:); Y];
    Vx0 = Last_Velocity_sim*cos(Last_Heading_sim);
    Vy0 = Last_Velocity_sim*sin(Last_Heading_sim);
    Yaw0 = Last_Heading_sim;
     
    T_sample = []; 
    for j = 1:length(X)
        T_sample = [T_sample; Tsim+(j-1)*Ts];
    end
    
   [Velocity_updated, Heading_updated] = P2YV(0, T_sample , X , Y , Vx0 , Vy0 , Yaw0, Np, Last_Heading_end );
   Heading_end = Heading_updated(end,:);

%     Heading_tmp_end = atan2(XYplot(end,2)-XYplot_sim(2,:), XYplot(end,1)-XYplot_sim(1,:));
% 
%     if  ((Heading_tmp_end - Heading_tmp_end_delay) < -5/3*pi) % Angle compensation
%         Heading_flag_end = Heading_flag_end + 1;
%     elseif ((Heading_tmp_end - Heading_tmp_end_delay) > 5/3*pi)
%         Heading_flag_end = Heading_flag_end - 1;
%     end
%     
%     if flag == 1
%         Heading_updated(1:end) = Heading_tmp_end + Heading_flag_end*2*pi;
%     end
%     if Tsim == 1.5
%         figure();
%         plot(XYplot(:,2),XYplot(:,1),'black-');
%         hold on;
%         plot(XYplot_sim(2,:),XYplot_sim(1,:),'b o');
%         plot(Veh_circle(:,2), Veh_circle(:,1),'b-');
%         plot(Veh_circle(:,4), Veh_circle(:,3),'b-');
%         plot(Veh_circle(:,6), Veh_circle(:,5),'b-');
%         plot(Veh_circle(:,8), Veh_circle(:,7),'b-');
%         plot(Veh_circle(:,10), Veh_circle(:,9),'b-');
%         plot(Y, X,'r x');
%     end

end

== matlab function Copy_of_MPC_control/all_system/Middle Observer2/Subsystem/VH2P/YV2P ==
  data: Velocity input; Yaw input; LastVelocity input; LastYaw input; Tsim input; LastTsim input; Lastpostion input; Position output
function Position  = YV2P(Velocity, Yaw,  LastVelocity, LastYaw, Tsim, LastTsim, Lastpostion)
if Tsim >= 0.1
    Position = zeros(2,1);
    X0 = Lastpostion(1,:); Y0 = Lastpostion(2,:);
    Vx = [LastVelocity*cos(LastYaw); Velocity*cos(Yaw)];
    Vy = [LastVelocity*sin(LastYaw); Velocity*sin(Yaw)];
    Yaw_sim = [LastYaw; Yaw];
    T_sample =[LastTsim; Tsim];
    [ X_tmp, Y_tmp] = YV2P( T_sample, X0, Y0, Vx, Vy, Yaw_sim, zeros(2,1) );
    Position = [X_tmp(end,:); Y_tmp(end,:)];
else
    Position = [0; 0];
end

end

== matlab function Copy_of_MPC_control/all_system/Middle Observer2/Subsystem/YV_update_Np/MATLAB Function2 ==
  data: XY_ref input; Velocity_updated output; XY_sim input; LastXY_sim input; Velocity_sim input; LastVelocity_sim input; Yaw_sim input; LastYaw_sim input; Tsim input; Heading_updated output
function [Velocity_updated, Heading_updated] = VY_update(XY_ref, XY_sim, LastXY_sim, Velocity_sim, LastVelocity_sim, Yaw_sim, LastYaw_sim, Tsim)
    disp(sprintf('Simulation time : %2.1f sec',Tsim)) 
 Ts = 0.1;
%  Np = 6;
 Np = 6;
 Heading_updated = zeros(Np,1); Velocity_updated = zeros(Np,1);
coder.extrinsic('P2YV');
% T_sample = [Tsim-0.01; Tsim; Tsim+0.01];
% X = [LastXY_sim(1); XY_sim(1); XY_ref(1,:)];
% Y = [LastXY_sim(2); XY_sim(2); XY_ref(2,:)];

% T_sample = [Tsim-0.01; Tsim; Tsim+0.01; Tsim+0.02];
% X = [LastXY_sim(1); XY_sim(1); XY_ref(1,:); XY_ref(3,:)];
% Y = [LastXY_sim(2); XY_sim(2); XY_ref(2,:); XY_ref(4,:)];

T_sample = []; 
for j = 1:Np+1
    T_sample = [T_sample; Tsim+(j-1)*Ts];
end
X = [];
for i = 1:Np
    X = [X; XY_ref(2*i-1,:)];
end
Y = [];
for i = 1:Np
    Y = [Y; XY_ref(2*i,:)];
end

X = [XY_sim(1,:); X];
Y = [XY_sim(2,:); Y];   
Vx0 = Velocity_sim*cos(Yaw_sim);
Vy0 = Velocity_sim*sin(Yaw_sim);
Yaw0 = Yaw_sim;

[Velocity_updated, Heading_updated] = P2YV(0,0, T_sample , X , Y , Vx0 , Vy0 , Yaw0, Np, 0, 0 );

end

== matlab function Copy_of_MPC_control/all_system/Middle_simulator1/Mpc_Simulator_Middle/MATLAB Function ==
  data: Ref output; JE input; U output; M input; Np input; phi input; Qc input; Fxh input; Yup input; Vup input; Rs input; Rs_V input; Tsim input; Upd_end input; u input; lambda output
function [Ref,U,lambda] = HQP(JE,M,Np,phi,Qc,Fxh,Yup,Vup,Rs,Rs_V,Tsim,Upd_end,u)

% if Tsim < 6.27 %(sec)
%     u1_max =  5/3*pi; u1_min = -5/3*pi;
%     u2_max =  0.3; u2_min = -1;
%     du1_inc =  1*5/3*pi; 
%     du1_dec =  1*5/3*pi; 
%     du2_inc =  0.03;
%     du2_dec =  0.03;
% else 
    u1_max =  5/3*pi; u1_min = -5/3*pi;
    u2_max =  1; u2_min = -1;
    du1_inc =  1*5/3*pi;
    du1_dec =  1*5/3*pi;
    du2_inc =  1;
    du2_dec =  1;
% end
% du1_max =  0.1*abs(Fxh(1,:)); 
% du2_max =  0.05*abs(Fxh(1,:)); 
% Y1_min = Rs(1,:) - 2;%V
% Y1_max = Rs(1,:) + 2;%V
% Y2_min = Rs(2,:) - 0.2;%Y
% Y2_max = Rs(2,:) + 0.2;%Y
% 
% Y1_min = -10;%V
% Y2_min = -100;%Y
% Y1_max = 50;%V
% Y2_max = 100;%Y

% Y_max = [];
% Y_min = [];
% for i = 1:Np
%     Y_max = [Y_max;[Y1_max;Y2_max]];
%     Y_min = [Y_min;[Y1_min;Y2_min]];
% end

U_max = []; U_min = [];
for i = 1:Np
    U_max = [U_max; [u1_max; u2_max]];
    U_min = [U_min; [-u1_min; -u2_min]];
end

dU_plus = []; dU_minus = [];
for i = 1:Np
    dU_plus = [dU_plus; [u(1) + du1_inc; u(2) + du2_inc]];
    dU_minus = [dU_minus; [-u(1) + du1_dec; -u(2) + du2_dec;]];
end
rr = [U_max;
      U_min;
      dU_plus;
      dU_minus;          
     ];
 
% rr_y = [Y_max - Fxh;
%        -Y_min + Fxh;
%        ];
N = [];
N = rr; 
% N = [rr;rr_y];

if Tsim > 0 && Tsim < Upd_end
    for i = 1: Np
        Rs(2*i,:) = Yup(i,:);
        Rs(2*i-1,:) = Vup(i,:);
    end
end

JF = -2*phi'*Qc*(Rs-Fxh);
[uc,lambda]= HQP(JE,JF,M,N);
U = uc(1:2);
Ref = Rs(1:2,:);
% lambda
end

== matlab function Copy_of_MPC_control/all_system/Middle_simulator1/VH2P/Trigger/Trigger ==
  data: timing input; Trigger output; Timetochange input
function Trigger = initial_position_trigger(timing,Timetochange)
Trigger = 0;    
    if timing == Timetochange
        Trigger = 1;
    end
end

== matlab function Copy_of_MPC_control/all_system/Middle_simulator1/VH2P/YV2P ==
  data: Velocity input; Yaw input; LastVelocity input; LastYaw input; Tsim input; LastTsim input; Lastpostion input; Position output
function Position  = YV2P(Velocity, Yaw,  LastVelocity, LastYaw, Tsim, LastTsim, Lastpostion)
if Tsim >= 0.1
    Position = zeros(2,1);
    X0 = Lastpostion(1,:); Y0 = Lastpostion(2,:);
    Vx = [LastVelocity*cos(LastYaw); Velocity*cos(Yaw)];
    Vy = [LastVelocity*sin(LastYaw); Velocity*sin(Yaw)];
    Yaw_sim = [LastYaw; Yaw];
    T_sample =[LastTsim; Tsim];
    [ X_tmp, Y_tmp] = YV2P( T_sample, X0, Y0, Vx, Vy, Yaw_sim, zeros(2,1) );
    Position = [X_tmp(end,:); Y_tmp(end,:)];
else
    Position = [0; 0];
end

end

== matlab function Copy_of_MPC_control/all_system/Middle_simulator1/YV_update_Np/MATLAB Function2 ==
  data: XY_ref input; Velocity_updated output; XY_sim input; LastXY_sim input; Velocity_sim input; LastVelocity_sim input; Yaw_sim input; LastYaw_sim input; Tsim input; Heading_updated output
function [Velocity_updated, Heading_updated] = VY_update(XY_ref, XY_sim, LastXY_sim, Velocity_sim, LastVelocity_sim, Yaw_sim, LastYaw_sim, Tsim)
    disp(sprintf('Simulation time : %2.1f sec',Tsim)) 
 Ts = 0.1;
%  Np = 6;
 Np = 6;

 Heading_updated = zeros(Np,1); Velocity_updated = zeros(Np,1);
coder.extrinsic('P2YV_Simulator');
% T_sample = [Tsim-0.01; Tsim; Tsim+0.01];
% X = [LastXY_sim(1); XY_sim(1); XY_ref(1,:)];
% Y = [LastXY_sim(2); XY_sim(2); XY_ref(2,:)];

% T_sample = [Tsim-0.01; Tsim; Tsim+0.01; Tsim+0.02];
% X = [LastXY_sim(1); XY_sim(1); XY_ref(1,:); XY_ref(3,:)];
% Y = [LastXY_sim(2); XY_sim(2); XY_ref(2,:); XY_ref(4,:)];

T_sample = []; 
for j = 1:Np+1
    T_sample = [T_sample; Tsim+(j-1)*Ts];
end
X = [];
for i = 1:Np
    X = [X; XY_ref(2*i-1,:)];
end
Y = [];
for i = 1:Np
    Y = [Y; XY_ref(2*i,:)];
end

X = [XY_sim(1,:); X];
Y = [XY_sim(2,:); Y];   
Vx0 = Velocity_sim*cos(Yaw_sim);
Vy0 = Velocity_sim*sin(Yaw_sim);
Yaw0 = Yaw_sim;

[Velocity_updated, Heading_updated] = P2YV_Simulator(0,0, T_sample , X , Y , Vx0 , Vy0 , Yaw0, Np, 0, 0 );

end

== matlab function Copy_of_MPC_control/all_system/Middle_simulator_ operating_time1/MATLAB Function2 ==
  data: timing input; state output; Timetochange input; Statechange2 input
function state = OperatingtimeMiddle(timing,Timetochange,Statechange2)
    if timing >= Timetochange && timing <= Statechange2
        state = 1;
    else
        state = 0;
    end
end

== matlab function Copy_of_MPC_control/all_system/Mpc_block1/Extrapolation_select/Select_model ==
  data: Time input; Select output; Tc1 input; Tc2 input
function Select = Extrapolation_select(Time, Tc1, Tc2)
    
if (Time >= Tc1 && Time < Tc1 + 1)
    Select = 1;
elseif Time > Tc2
    Select = 1;
else 
    Select = 0;
end

end

== matlab function Copy_of_MPC_control/all_system/Mpc_block1/Mpc ==
  data: Upd_flag input; JE input; Timetochange input; Timetochange2 input; Ts input; U output; Ref output; lambda output; u1 output; M input; Np input; JF_part input; U_min input; U_max input; Fxh input; Rs_Y input; Rs_V input; Yup input [1..5]; Vup input [1..5]; Rs input; Tsim input; Upd_end input; u input; u1 input; u2 input; u3 input; u2 output; u3 output
function [U, Ref, lambda, u1, u2, u3] = HQP(Upd_flag, JE, Timetochange, Timetochange2, Ts, M, Np, JF_part, U_min, U_max, Fxh, Rs_Y, Rs_V, Yup, Vup, Rs, Tsim,Upd_end, u, u1, u2, u3)
Ue = zeros(2,1); U = zeros(2,1);
% coder.varsize('Vup', [5 1]);
% disp(sprintf('Simulation time : %2.2f sec',Tsim)) 
% if (Tsim==0)
%     plot(XYplot(:,2),XYplot(:,1));
% end
% if Tsim > 68 %(sec)
%     u1_max =  5/3*pi; u1_min = -5/3*pi;
%     u1_max =  -1; u1_min = -1.05;
%     u2_max =  -0.1; u2_min = -0.12;
%     du1_inc =  0.005*5/3*pi; 
%     du1_dec =  0.005*5/3*pi; 
%     du2_inc =  0.005;
%     du2_dec =  0.005;
% else 

    du1_inc = 1*5/3*pi;
    du1_dec = 1*5/3*pi;
    du2_inc = 1;
    du2_dec = 1;
%     du2_inc = 0.64;
%     du2_dec = 0.64;
% end
% du1_max =  0.1*abs(Fxh(1,:)); 
% du2_max =  0.05*abs(Fxh(1,:)); 
% Y1_min = Rs(1,:) - 2;%V
% Y1_max = Rs(1,:) + 2;%V
% Y2_min = Rs(2,:) - 0.2;%Y
% Y2_max = Rs(2,:) + 0.2;%Y
% 
% Y1_min = -10;%V
% Y2_min = -100;%Y
% Y1_max = 50;%V
% Y2_max = 100;%Y

% Y_max = [];
% Y_min = [];
% for i = 1:Np
%     Y_max = [Y_max;[Y1_max;Y2_max]];
%     Y_min = [Y_min;[Y1_min;Y2_min]];
% end

% U_max = []; U_min = [];
% for i = 1:Np
%     U_max = [U_max; [u1_max; u2_max]];
%     U_min = [U_min; [-u1_min; -u2_min]];
% end

dU_plus = []; dU_minus = [];
for i = 1:Np
    dU_plus = [dU_plus; [u(1) + du1_inc; u(2) + du2_inc]];
    dU_minus = [dU_minus; [-u(1) + du1_dec; -u(2) + du2_dec;]];
end
rr = [U_max;
      U_min;
      dU_plus;
      dU_minus;          
     ];
 
% rr_y = [Y_max - Fxh;
%        -Y_min + Fxh;
%        ];
N = [];
N = rr; 
% N = [rr;rr_y];
% if Tsim > 0.1
%     Rs = [];
%     for i = 1:Np
%         Rs = [Rs; Rs_V(i,:); Yup(i,:)];
%     end
% else 
%     Rs = [];
%     for i = 1:Np
%         Rs = [Rs; Rs_V(i,:); Rs_Y(i,:)];
%     end
% end

% Rs = [];
% for i = 1:Np
%     Rs = [Rs; Rs_V(i,:); Rs_heading_angle];
% end
% 

if Tsim > 0 && Tsim < Upd_end
    for i = 1: Np
        Rs(2*i,:) = Yup(i,:);
        Rs(2*i-1,:) = Vup(i,:);
    end
end


JF = JF_part*(Rs-Fxh);
[uc,lambda]= HQP(JE,JF,M,N);
un = uc(1:2);

% Extrapolation

% if (Tsim >= Timetochange && Tsim < Timetochange + 0.5)
%     
%     pp = [0 0 1; Ts^2 Ts 1; 4*Ts^2 2*Ts 1];
%     vv = [u3(1,:); u2(1,:); u1(1,:)];
%     abc = inv(pp)*vv;
%     Ue(1,:) = polyval(abc,((Tsim-Timetochange)/Ts+2)*Ts);
%     vv = [u3(2,:); u2(2,:); u1(2,:)];
%     abc = inv(pp)*vv;
%     Ue(2,:) = polyval(abc,((Tsim-Timetochange)/Ts+2)*Ts);
%     U = Ue;
% elseif (Tsim >= Timetochange2 && Tsim < Timetochange2 + 1)
%     
%     pp = [0 0 1; Ts^2 Ts 1; 4*Ts^2 2*Ts 1];
%     vv = [u3(1,:); u2(1,:); u1(1,:)];
%     abc = inv(pp)*vv;
%     Ue(1,:) = polyval(abc,((Tsim-Timetochange2)/Ts+2)*Ts);
%     vv = [u3(2,:); u2(2,:); u1(2,:)];
%     abc = inv(pp)*vv;
%     Ue(2,:) = polyval(abc,((Tsim-Timetochange2)/Ts+2)*Ts);
%     U = Ue;
% else
%     U = un;
% end
U = un;
% if Tsim <= Timetochange
%     U(1,:) = 1e-9;
% end
Ref = Rs(1:2,:);
% lambda
end

== matlab function Copy_of_MPC_control/all_system/Observer_state1/Observer_state1 ==
  data: timing input; state output; point input
function state = Observer_state1(timing,point)
    if timing > point
        state = 0;
    else
        state = 1;
    end
end

== matlab function Copy_of_MPC_control/all_system/Observer_state2/Observer_state2 ==
  data: timing input; state output; Earlytochange input; Timetochange2 input
function state = Observer_state2(timing,Earlytochange,Timetochange2)
    if timing >= Earlytochange && timing <= Timetochange2
        state = 1;
    else
        state = 0;
    end
end

== matlab function Copy_of_MPC_control/all_system/Observer_state3/Observer_state2 ==
  data: timing input; state output; Earlytochange2 input
function state = Observer_state2(timing,Earlytochange2)
    if timing >= Earlytochange2
        state = 1;
    else
        state = 0;
    end
end

== matlab function Copy_of_MPC_control/all_system/Passenger Vehicle1/beta ==
  data: beta output; ydot input; Velocity output; xdot input
function [beta, Velocity]  = Velocity(ydot, xdot)
beta = 0; Velocity = 0;
Velocity = sqrt(xdot^2 + ydot^2);

xdot = abs(xdot);

beta = atan2(ydot, xdot);
end

== matlab function Copy_of_MPC_control/all_system/Select_model1/Select_model ==
  data: Time input; Select output; Tc1 input; Tc2 input
function Select = Select_model(Time, Tc1, Tc2)
    disp(sprintf('Simulation time : %2.1f sec',Time)) 

if (Time < Tc1)
    Select = 1;
elseif (Time < Tc2)
    Select = 2;
elseif (Time >= Tc2)
    Select = 3;
else
    Select = 4;
end

end

== matlab function Copy_of_MPC_control/all_system/Subsystem2/Dataselect/Dataselect ==
  data: timing input; select output; Statechange input; Statechange2 input
function select = Dataselect(timing,Statechange,Statechange2)    
    if timing < Statechange
        select = 1;
    elseif timing < Statechange2
        select = 2;
    else 
        select = 3;
    end
end
